simulink model "EV3_terme_integral"  (R2025b)
settings: Solver=FixedStepAuto  StartTime=0.0  StopTime=10.0  RelTol=1e-3  EnableMultiTasking=on
values from neighbouring files (symbols this model uses):
  A_1 = [zeros(2) eye(2) ... (first row only)    [model.m]
  B_1 = [0;0 ... (first row only)    [model.m]
  gamma = 0.999    [model.m]
  H_barre = K_t(5)    [model.m]
  K_int = K_t(1:4)    [model.m]
  K_PWM = 8.087    [model.m]
  Psi0 = deg2rad(8)    [model.m]
  s1 = ss(A_1, B_1, eye(4), zeros(4,1))    [model.m]
  Ts = 0.004    [model.m]
undefined symbols (not defined in the file or in its folder): DiscIntNeverNeededParam
libraries: legoev3lib x5, simulink x2
settings Model: ExtModeTrigDuration=2  Creator=carol  LastModifiedBy=carol
settings SolverCC: PositivePriorityOrder=on
settings OptimizationCC: DefaultParameterBehavior=Inlined  EnhancedBackFolding=on  PassReuseOutputArgsAs=Individual arguments  ZeroExternalMemoryAtStartup=off  ZeroInternalMemoryAtStartup=off  MaxStackSize=64  OptimizeBlockOrder=speed  DifferentSizesBufferReuse=on  OptimizationCustomize=off  EfficientTunableParamExpr=on
settings DebuggingCC: ParameterTunabilityLossMsg=error
settings HardwareCC: ProdBitPerPointer=32.0  ProdBitPerSizeT=32.0  ProdBitPerPtrDiffT=32.0  ProdLargestAtomicInteger=Long  ProdWordSize=32.0  ProdHWDeviceType=ARM Compatible->ARM 9  UseEmbeddedCoderFeatures=off  UseSimulinkCoderFeatures=off
settings SFSimCC: MATLABDynamicMemAlloc=off
settings RTWCC: SystemTargetFile=ert.tlc  HardwareBoard=LEGO MINDSTORMS EV3  TLCOptions="-aInlineSetEventsForThisBaseRateFcn=TLC_FALSE -aSuppressMultiTaskScheduler=TLC_FALSE  -aRateBasedStepFcn=0"  TemplateMakefile=ert_default_tmf  Toolchain=Sourcery G++ Lite v2009q3  Description=Embedded Coder
settings CodeAppCC: ForceParamTrailComments=on  IgnoreCustomStorageClasses=off  OperatorAnnotations=on  SimulinkDataObjDesc=on  SFDataObjDesc=on  InsertBlockDesc=on
settings ERTTargetCC: ExtModeTransport=2.0  ExtModeStaticAlloc=on  ExtModeMexFile=ext_xcp  ExtModeIntrfLevel=Level2 - Open  SupportContinuousTime=on  SupportNonInlinedSFcns=on  SupportVariableSizeSignals=on

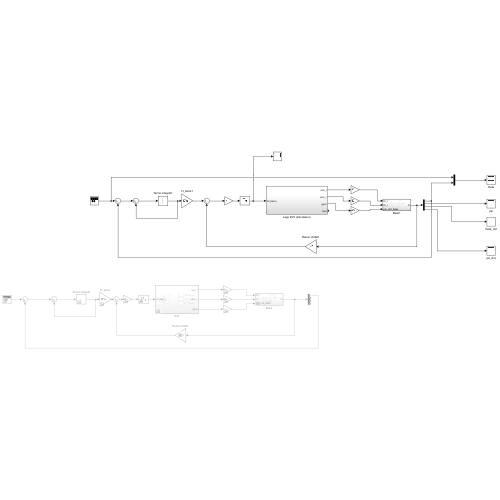
[thumbnail: Simulink's stored preview of the top-level diagram]
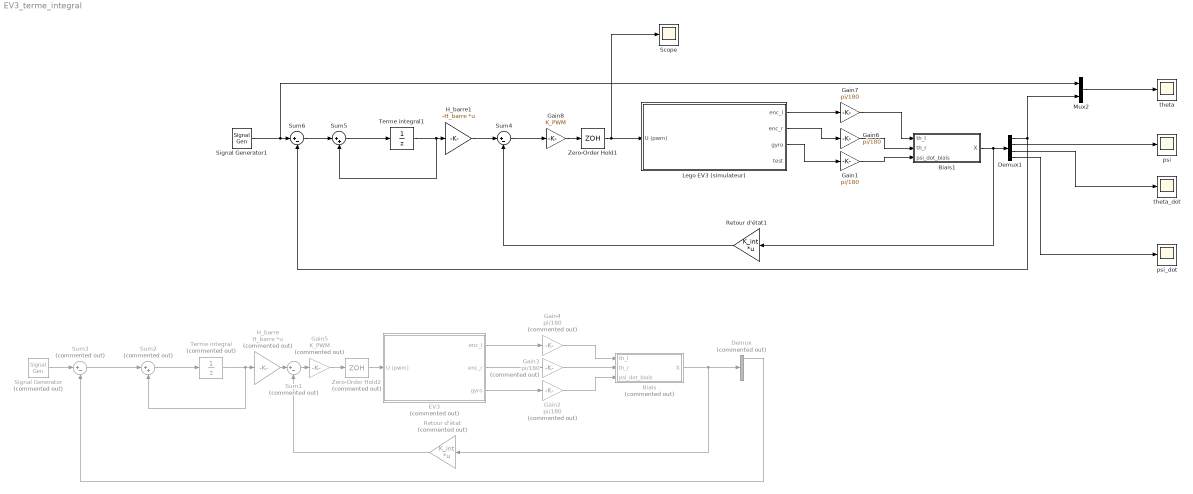
== system EV3_terme_integral ==
  Biais : Subsystem  Commented=on
  Biais1 : Subsystem
  Demux : Demux  Commented=on
  Demux1 : Demux
  EV3 : Subsystem  Commented=on
  Gain1 : Gain  Gain=pi/180
  Gain2 : Gain  Commented=on  Gain=pi/180
  Gain3 : Gain  Commented=on  Gain=pi/180
  Gain4 : Gain  Commented=on  Gain=pi/180
  Gain5 : Gain  Commented=on  Gain=K_PWM
  Gain6 : Gain  Gain=pi/180
  Gain7 : Gain  Gain=pi/180
  Gain8 : Gain  Gain=K_PWM
  H_barre : Gain  Commented=on  Gain=H_barre  Multiplication=Matrix(K*u)
  H_barre1 : Gain  Gain=-H_barre  Multiplication=Matrix(K*u)
  Lego EV3 (simulateur) : Subsystem
  Mux2 : Mux  Inputs=2
  Retour d'état : Gain  Commented=on  Gain=K_int  Multiplication=Matrix(K*u)
  Retour d'état1 : Gain  Gain=K_int  Multiplication=Matrix(K*u)
  Scope : Scope
      settings: ActiveDisplayYMinimum=-623.65580691886532  ActiveDisplayYMaximum=405.37809192653361  DataLoggingVariableName=ScopeData11
  Signal Generator : SignalGenerator  Commented=on  WaveForm=square  Amplitude=0  Frequency=0.1
  Signal Generator1 : SignalGenerator  WaveForm=square  Amplitude=0  Frequency=0.1
  Sum1 : Sum  Commented=on  Inputs=|+-
  Sum2 : Sum  Commented=on  Inputs=|++
  Sum3 : Sum  Commented=on  Inputs=|+-
  Sum4 : Sum  Inputs=|+-
  Sum5 : Sum  Inputs=|++
  Sum6 : Sum  Inputs=|+-
  Terme integral : UnitDelay  Commented=on  SampleTime=-1  HasFrameUpgradeWarning=on
  Terme integral1 : UnitDelay  SampleTime=-1  HasFrameUpgradeWarning=on
  Zero-Order Hold1 : ZeroOrderHold  SampleTime=Ts
  Zero-Order Hold2 : ZeroOrderHold  Commented=on  SampleTime=Ts
  psi : Scope
      settings: ActiveDisplayYMinimum=-1  ActiveDisplayYMaximum=1  DataLoggingVariableName=ScopeData5
  psi_dot : Scope
      settings: ActiveDisplayYMinimum=-4.9328102341799545  ActiveDisplayYMaximum=4.93528931485691  DataLoggingVariableName=ScopeData7
  theta : Scope
      settings: ActiveDisplayYMinimum=-8.7269371878959834E+28  ActiveDisplayYMaximum=9.69659687543998E+27  DataLoggingVariableName=ScopeData4
  theta_dot : Scope
      settings: ActiveDisplayYMinimum=-1  ActiveDisplayYMaximum=1  DataLoggingVariableName=ScopeData6
  wires:
  EV3/3(gyro) -> Gain2/1
  Gain4/1 -> Biais/1(th_l)
  Biais/1(X) -> Retour d'état/1, Demux/1
  EV3/1(enc_l) -> Gain4/1
  Gain3/1 -> Biais/2(th_r)
  Gain2/1 -> Biais/3(psi_dot_biais)
  EV3/2(enc_r) -> Gain3/1
  Sum1/1 -> Gain5/1
  Zero-Order Hold2/1 -> EV3/1(U (pwm))
  Gain5/1 -> Zero-Order Hold2/1
  Retour d'état/1 -> Sum1/2
  Terme integral/1 -> Sum2/2, H_barre/1
  H_barre/1 -> Sum1/1
  Sum2/1 -> Terme integral/1
  Sum3/1 -> Sum2/1
  Signal Generator/1 -> Sum3/1
  Demux/1 -> Sum3/2
  Demux1/4 -> psi_dot/1
  Zero-Order Hold1/1 -> Lego EV3 (simulateur)/1(U (pwm)), Scope/1
  Lego EV3 (simulateur)/2(enc_r) -> Gain6/1
  Demux1/2 -> psi/1
  Gain8/1 -> Zero-Order Hold1/1
  Gain6/1 -> Biais1/2(th_r)
  Lego EV3 (simulateur)/1(enc_l) -> Gain7/1
  Sum4/1 -> Gain8/1
  Retour d'état1/1 -> Sum4/2
  Biais1/1(X) -> Retour d'état1/1, Demux1/1
  Lego EV3 (simulateur)/3(gyro) -> Gain1/1
  Gain1/1 -> Biais1/3(psi_dot_biais)
  Demux1/3 -> theta_dot/1
  Mux2/1 -> theta/1
  Gain7/1 -> Biais1/1(th_l)
  Sum6/1 -> Sum5/1
  Demux1/1 -> Mux2/2, Sum6/2
  Terme integral1/1 -> Sum5/2, H_barre1/1
  Sum5/1 -> Terme integral1/1
  H_barre1/1 -> Sum4/1
  Signal Generator1/1 -> Mux2/1, Sum6/1

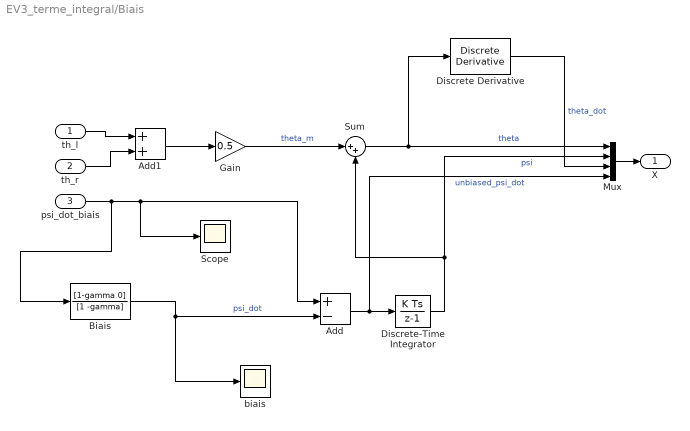
== system EV3_terme_integral/Biais ==
  th_l : Inport
  th_r : Inport  Port=2
  psi_dot_biais : Inport  Port=3
  Add : Sum  Inputs=+-
  Add1 : Sum
  Biais : DiscreteTransferFcn  Numerator=[1-gamma 0]  Denominator=[1 -gamma]
  Discrete Derivative : simulink/Quick Insert/Discrete/Discrete Derivative  gainval=1.0  ICPrevScaledInput=0.0  OutMin=[]  OutMax=[]  OutDataType=fixdt(1, 16)  OutScaling=2^-10  DoSatur=off
  Discrete-Time Integrator : DiscreteIntegrator  SampleTime=Ts  ICPrevOutput=DiscIntNeverNeededParam  ICPrevScaledInput=DiscIntNeverNeededParam
  Gain : Gain  Gain=0.5
  Mux : Mux
  Scope : Scope
      settings: ActiveDisplayYMinimum=-1  ActiveDisplayYMaximum=1  DataLoggingVariableName=ScopeData13
  Sum : Sum  Inputs=|++
  biais : Scope
      settings: ActiveDisplayYMinimum=-0.1164059395354744  ActiveDisplayYMaximum=0.0646369691442869  DataLoggingVariableName=ScopeData12
  X : Outport
  wires:
  th_l/1 -> Add1/1
  th_r/1 -> Add1/2
  Add1/1 -> Gain/1
  Mux/1 -> X/1
  Discrete Derivative/1 -> Mux/3  "theta_dot"
  Discrete-Time Integrator/1 -> Sum/2, Mux/2  "psi"
  psi_dot_biais/1 -> Biais/1, Scope/1, Add/1
  Biais/1 -> Add/2, biais/1  "psi_dot"
  Add/1 -> Mux/4, Discrete-Time Integrator/1  "unbiased_psi_dot"
  Gain/1 -> Sum/1  "theta_m"
  Sum/1 -> Mux/1, Discrete Derivative/1  "theta"

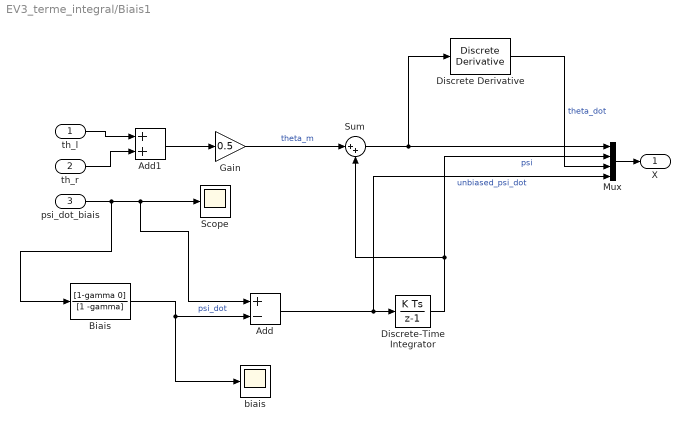
== system EV3_terme_integral/Biais1 ==
  th_l : Inport
  th_r : Inport  Port=2
  psi_dot_biais : Inport  Port=3
  Add : Sum  Inputs=+-
  Add1 : Sum
  Biais : DiscreteTransferFcn  Numerator=[1-gamma 0]  Denominator=[1 -gamma]
  Discrete Derivative : simulink/Quick Insert/Discrete/Discrete Derivative  gainval=1.0  ICPrevScaledInput=0.0  OutMin=[]  OutMax=[]  OutDataType=fixdt(1, 16)  OutScaling=2^-10  DoSatur=off
  Discrete-Time Integrator : DiscreteIntegrator  SampleTime=Ts  ICPrevOutput=DiscIntNeverNeededParam  ICPrevScaledInput=DiscIntNeverNeededParam
  Gain : Gain  Gain=0.5
  Mux : Mux
  Scope : Scope
      settings: ActiveDisplayYMinimum=-1  ActiveDisplayYMaximum=1  DataLoggingVariableName=ScopeData13
  Sum : Sum  Inputs=|++
  biais : Scope
      settings: ActiveDisplayYMinimum=-0.1164059395354744  ActiveDisplayYMaximum=0.0646369691442869  DataLoggingVariableName=ScopeData12
  X : Outport
  wires:
  th_l/1 -> Add1/1
  th_r/1 -> Add1/2
  Add1/1 -> Gain/1
  Mux/1 -> X/1
  Discrete Derivative/1 -> Mux/3  "theta_dot"
  Discrete-Time Integrator/1 -> Sum/2, Mux/2  "psi"
  psi_dot_biais/1 -> Biais/1, Add/1, Scope/1
  Biais/1 -> Add/2, biais/1  "psi_dot"
  Add/1 -> Mux/4, Discrete-Time Integrator/1  "unbiased_psi_dot"
  Gain/1 -> Sum/1  "theta_m"
  Sum/1 -> Mux/1, Discrete Derivative/1

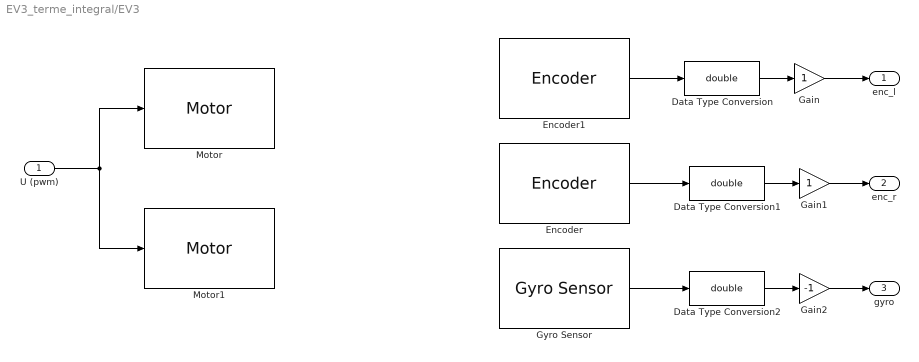
== system EV3_terme_integral/EV3 ==
  U (pwm) : Inport
  Data Type Conversion : DataTypeConversion  OutDataTypeStr=double  SaturateOnIntegerOverflow=off  RndMeth=Floor
  Data Type Conversion1 : DataTypeConversion  OutDataTypeStr=double  SaturateOnIntegerOverflow=off  RndMeth=Floor
  Data Type Conversion2 : DataTypeConversion  OutDataTypeStr=double  SaturateOnIntegerOverflow=off  RndMeth=Floor
  Encoder : legoev3lib/Encoder  portNumber=A  opMode=Reset by external signal  sampleTime=Ts
  Encoder1 : legoev3lib/Encoder  portNumber=D  opMode=Reset by external signal  sampleTime=Ts
  Gain : Gain
  Gain1 : Gain
  Gain2 : Gain  Gain=-1
  Gyro Sensor : legoev3lib/Gyro Sensor  portNumber=3  sampleTime=Ts
  Motor : legoev3lib/Motor  sportNumber=D  sstopAction=Brake
  Motor1 : legoev3lib/Motor  sportNumber=A  sstopAction=Brake
  enc_l : Outport
  enc_r : Outport  Port=2
  gyro : Outport  Port=3
  wires:
  Gyro Sensor/1 -> Data Type Conversion2/1
  Encoder/1 -> Data Type Conversion1/1
  Encoder1/1 -> Data Type Conversion/1
  Data Type Conversion/1 -> Gain/1
  Data Type Conversion1/1 -> Gain1/1
  Data Type Conversion2/1 -> Gain2/1
  U (pwm)/1 -> Motor1/1, Motor/1
  Gain/1 -> enc_l/1
  Gain1/1 -> enc_r/1
  Gain2/1 -> gyro/1

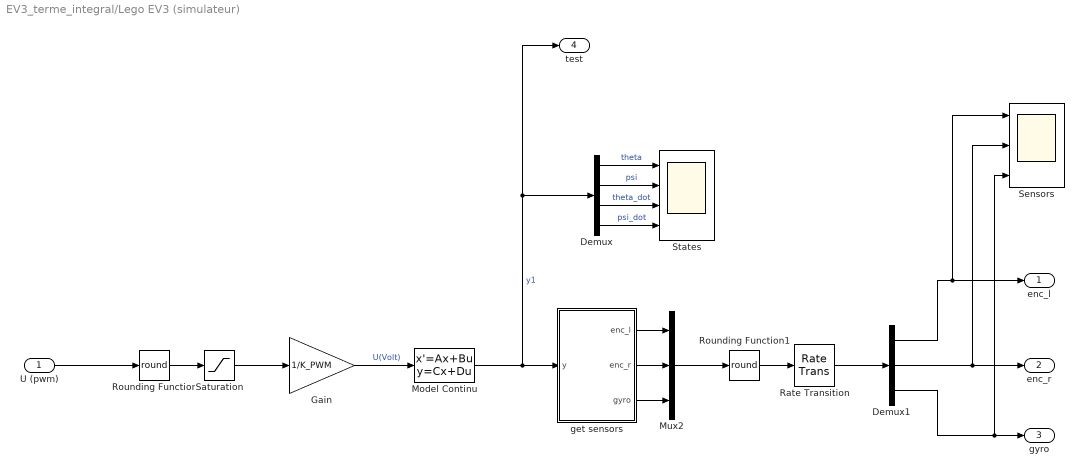
== system EV3_terme_integral/Lego EV3 (simulateur) ==
  U (pwm) : Inport
  Demux : Demux
  Demux1 : Demux  Outputs=3
  Gain : Gain  Gain=1/K_PWM
  Model Continu : StateSpace  A=A_1  B=B_1  C=eye(4)  D=s1.D  InitialCondition=[0 Psi0 0 0]
  Mux2 : Mux  Inputs=3
  Rate Transition : RateTransition  OutPortSampleTime=Ts
  Rounding Function : Rounding  Operator=round
  Rounding Function1 : Rounding  Operator=round
  Saturation : Saturate  UpperLimit=100  LowerLimit=-100
  Sensors : Scope  NumInputPorts=3
      settings: ActiveDisplayYMinimum=-115  ActiveDisplayYMaximum=265
  States : Scope  NumInputPorts=4
      settings: ActiveDisplayYMinimum=-18.762173178074935  ActiveDisplayYMaximum=8.1937673053565856  DataLoggingVariableName=ScopeData2
  get sensors : MATLAB Function  TreatAsAtomicUnit=on
  enc_l : Outport
  enc_r : Outport  Port=2
  gyro : Outport  Port=3
  test : Outport  Port=4
  wires:
  Model Continu/1 -> test/1, Demux/1, get sensors/1(y)  "y1"
  Gain/1 -> Model Continu/1  "U(Volt)"
  Saturation/1 -> Gain/1
  U (pwm)/1 -> Rounding Function/1
  get sensors/3(gyro) -> Mux2/3
  Demux/4 -> States/4  "psi_dot"
  Rounding Function1/1 -> Rate Transition/1
  Demux/2 -> States/2  "psi"
  Demux/3 -> States/3  "theta_dot"
  Demux/1 -> States/1  "theta"
  get sensors/1(enc_l) -> Mux2/1
  get sensors/2(enc_r) -> Mux2/2
  Rounding Function/1 -> Saturation/1
  Mux2/1 -> Rounding Function1/1
  Rate Transition/1 -> Demux1/1
  Demux1/1 -> Sensors/1, enc_l/1
  Demux1/2 -> Sensors/2, enc_r/1
  Demux1/3 -> Sensors/3, gyro/1

== matlab function EV3_terme_integral/Lego EV3 (simulateur)/get sensors ==
  data: enc_l output; enc_r output; y input; gyro output; R parameter
function [enc_l, enc_r, gyro] = sensors(y, R)
enc_l = rad2deg(y(1) - y(2));
enc_r = rad2deg(y(1) - y(2));
gyro  = rad2deg(y(4));
